simulink model "PCC_Calibration_Simu"  (R2015b)
settings: Solver=ode3  StartTime=0.0  StopTime=1373  FixedStep=0.01  RelTol=1e-3
model workspace: external: MAT-File params.mat (data not in the file)
undefined symbols (not defined in the file): aeroDragCoeff, airDensity, discIntervalf, discIntervals, DiscIntNeverNeededParam, FD, frontArea, G1, G2, G3, G4, G5, G6, gravity, inertialMassVeh, iterNum, lambdaRange, magnitude, massVeh, MDL, powerWeif, powerWeis, predPeriodf, predPeriods, rollingResistCoeff, terminThreshold, terminTimedis, terminVeloweif, terminVeloweis, wheelRadius, z_ACCe
libraries: simulink x16
(part 1 of 5)
settings Model: Creator=yanyongjun  LastModifiedBy=Administrator
settings DataIOCC: SaveFormat=Array
settings DebuggingCC: UnderspecifiedInitializationDetection=Classic  MergeDetectMultiDrivingBlocksExec=none  SolverPrmCheckMsg=warning  MultiTaskCondExecSysMsg=warning  MultiTaskRateTransMsg=warning
settings HardwareCC: ProdBitPerPointer=32  ProdLargestAtomicFloat=None  ProdIntDivRoundTo=Undefined  ProdEndianess=Unspecified  ProdWordSize=32  ProdHWDeviceType=32-bit Generic
settings GRTTargetCC: GeneratePreprocessorConditionals=Disable all
settings ConfigComp: CovModelRefEnable=Off

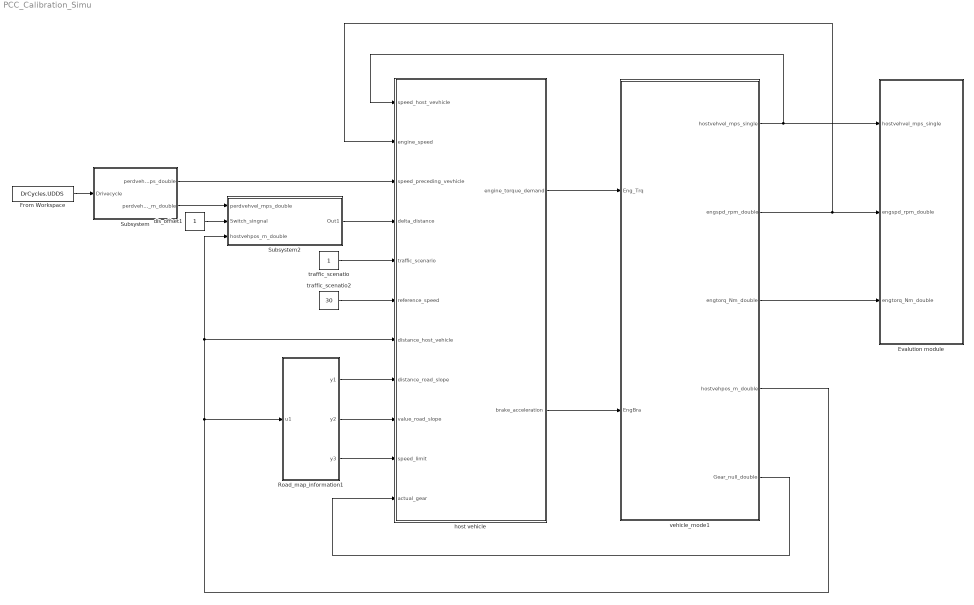
== system PCC_Calibration_Simu ==
  Evalution module : Subsystem
  From Workspace : FromWorkspace  VariableName=DrCycles.UDDS  SampleTime=0.01
  Road_map_information1 : MATLAB Function  TreatAsAtomicUnit=on
  Subsystem : Subsystem
  Subsystem2 : Subsystem
  dis_offset1 : Constant  OutDataTypeStr=double
  host vehicle : Subsystem
  traffic_scenatio : Constant  OutDataTypeStr=double
  traffic_scenatio2 : Constant  Value=30  OutDataTypeStr=double
  vehicle_mode1 : Subsystem
  wires:
  traffic_scenatio/1 -> host vehicle/5(traffic_scenario)
  Subsystem2/1(Out1) -> host vehicle/4(delta_distance)
  Subsystem/1(perdvehvel_mps_double) -> host vehicle/3(speed_preceding_vevhicle)
  traffic_scenatio2/1 -> host vehicle/6(reference_speed)
  vehicle_mode1/4(hostvehpos_m_double) -> Subsystem2/3(hostvehpos_m_double), host vehicle/7(distance_host_vehicle), Road_map_information1/1(u1)
  Road_map_information1/3(y3) -> host vehicle/10(speed_limit)
  Road_map_information1/2(y2) -> host vehicle/9(value_road_slope)
  host vehicle/1(engine_torque_demand) -> vehicle_mode1/1(Eng_Trq)
  Road_map_information1/1(y1) -> host vehicle/8(distance_road_slope)
  host vehicle/2(brake_acceleration) -> vehicle_mode1/2(EngBra)
  vehicle_mode1/5(Gear_null_double) -> host vehicle/11(actual_gear)
  vehicle_mode1/1(hostvehvel_mps_single) -> host vehicle/1(speed_host_vevhicle), Evalution module/1(hostvehvel_mps_single)
  From Workspace/1 -> Subsystem/1(Drivecycle)
  vehicle_mode1/3(engtorq_Nm_double) -> Evalution module/3(engtorq_Nm_double)
  Subsystem/2(perdvehpos_m_double) -> Subsystem2/1(perdvehvel_mps_double)
  dis_offset1/1 -> Subsystem2/2(Switch_singnal)
  vehicle_mode1/2(engspd_rpm_double) -> host vehicle/2(engine_speed), Evalution module/2(engspd_rpm_double)

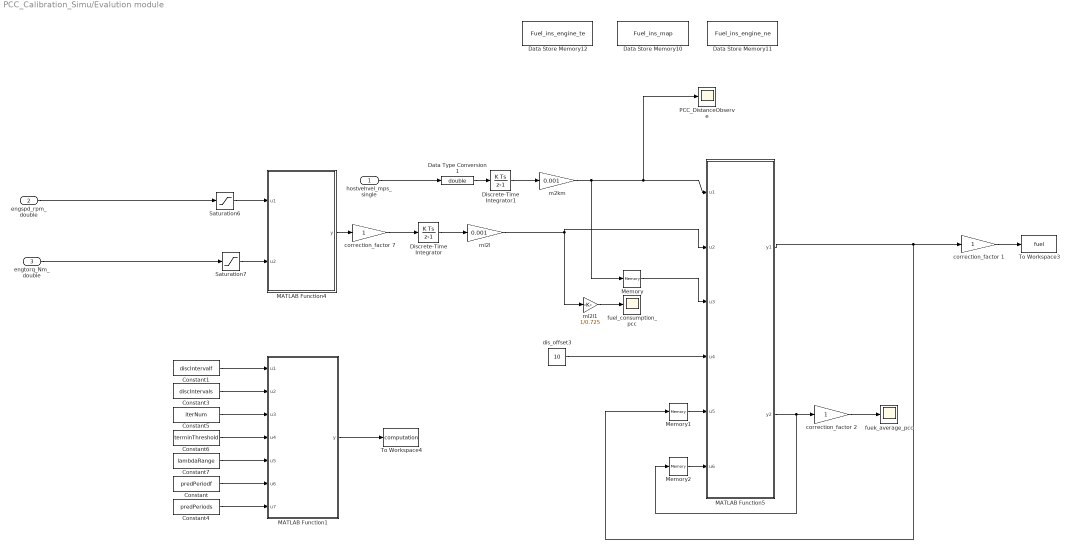
== system PCC_Calibration_Simu/Evalution module ==
  hostvehvel_mps_single : Inport
  engspd_rpm_double : Inport  Port=2
  engtorq_Nm_double : Inport  Port=3
  " ml2l" : Gain  Gain=0.001  SampleTime=0.01
  " ml2l1" : Gain  Gain=1/0.725  SampleTime=0.01
  Constant : Constant  Value=predPeriodf  OutDataTypeStr=double  SampleTime=0.01
  Constant1 : Constant  Value=discIntervalf  OutDataTypeStr=double  SampleTime=0.01
  Constant3 : Constant  Value=discIntervals  OutDataTypeStr=double  SampleTime=0.01
  Constant4 : Constant  Value=predPeriods  OutDataTypeStr=double  SampleTime=0.01
  Constant5 : Constant  Value=iterNum  OutDataTypeStr=double  SampleTime=0.01
  Constant6 : Constant  Value=terminThreshold  OutDataTypeStr=double  SampleTime=0.01
  Constant7 : Constant  Value=lambdaRange  OutDataTypeStr=double  SampleTime=0.01
  Data Store Memory10 : DataStoreMemory  DataStoreName=Fuel_ins_map  InitialValue=ones(21,111)  OutDataTypeStr=double
  Data Store Memory11 : DataStoreMemory  DataStoreName=Fuel_ins_engine_ne  InitialValue=ones(21,111)  OutDataTypeStr=double
  Data Store Memory12 : DataStoreMemory  DataStoreName=Fuel_ins_engine_te  InitialValue=ones(21,111)  OutDataTypeStr=double
  Data Type Conversion1 : DataTypeConversion  OutDataTypeStr=double
  Discrete-Time Integrator : DiscreteIntegrator  SampleTime=0.01  ICPrevOutput=DiscIntNeverNeededParam  ICPrevScaledInput=DiscIntNeverNeededParam
  Discrete-Time Integrator1 : DiscreteIntegrator  SampleTime=0.01  ICPrevOutput=DiscIntNeverNeededParam  ICPrevScaledInput=DiscIntNeverNeededParam
  MATLAB Function1 : MATLAB Function  TreatAsAtomicUnit=on
  MATLAB Function4 : MATLAB Function  TreatAsAtomicUnit=on
  MATLAB Function5 : MATLAB Function  TreatAsAtomicUnit=on
  Memory : Memory
  Memory1 : Memory
  Memory2 : Memory
  PCC_DistanceObserve : Scope
  Saturation6 : Saturate  UpperLimit=6500  LowerLimit=700
  Saturation7 : Saturate  UpperLimit=200  LowerLimit=-40
  To Workspace3 : ToWorkspace  VariableName=fuel  SampleTime=-1
  To Workspace4 : ToWorkspace  VariableName=computation  SampleTime=-1
  correction_factor 1 : Gain  SampleTime=0.01
  correction_factor 2 : Gain  SampleTime=0.01
  correction_factor 7 : Gain  SampleTime=0.01
  dis_offset3 : Constant  Value=10  OutDataTypeStr=double
  fuek_average_pcc : Scope
  fuel_consumption_pcc : Scope
  m2km : Gain  Gain=0.001  SampleTime=0.01
  wires:
  MATLAB Function5/1(y1) -> Memory1/1, correction_factor 1/1
  Memory/1 -> MATLAB Function5/3(u3)
  " ml2l"/1 -> MATLAB Function5/2(u2), " ml2l1"/1
  dis_offset3/1 -> MATLAB Function5/4(u4)
  Memory1/1 -> MATLAB Function5/5(u5)
  Memory2/1 -> MATLAB Function5/6(u6)
  m2km/1 -> Memory/1, PCC_DistanceObserve/1, MATLAB Function5/1(u1)
  engtorq_Nm_double/1 -> Saturation7/1
  correction_factor 1/1 -> To Workspace3/1
  Data Type Conversion1/1 -> Discrete-Time Integrator1/1
  MATLAB Function5/2(y2) -> Memory2/1, correction_factor 2/1
  hostvehvel_mps_single/1 -> Data Type Conversion1/1
  MATLAB Function4/1(y) -> correction_factor 7/1
  Discrete-Time Integrator/1 -> " ml2l"/1
  correction_factor 2/1 -> fuek_average_pcc/1
  Saturation6/1 -> MATLAB Function4/1(u1)
  correction_factor 7/1 -> Discrete-Time Integrator/1
  Discrete-Time Integrator1/1 -> m2km/1
  " ml2l1"/1 -> fuel_consumption_pcc/1
  Saturation7/1 -> MATLAB Function4/2(u2)
  engspd_rpm_double/1 -> Saturation6/1
  Constant1/1 -> MATLAB Function1/1(u1)
  MATLAB Function1/1(y) -> To Workspace4/1
  Constant5/1 -> MATLAB Function1/3(u3)
  Constant6/1 -> MATLAB Function1/4(u4)
  Constant7/1 -> MATLAB Function1/5(u5)
  Constant3/1 -> MATLAB Function1/2(u2)
  Constant/1 -> MATLAB Function1/6(u6)
  Constant4/1 -> MATLAB Function1/7(u7)

== system PCC_Calibration_Simu/Subsystem ==
  Drivecycle : Inport
  Add : Sum  Inputs=+-
  PID Controller : simulink/Continuous/PID Controller  Controller=PID  TimeDomain=Discrete-time  SampleTime=-1  IntegratorMethod=Forward Euler  FilterMethod=Forward Euler  Form=Parallel  UseFilter=on  ControllerParametersSource=internal  P=6  I=1  D=0  N=100  InitialConditionSource=internal  InitialConditionForIntegrator=0  InitialConditionForFilter=0  ExternalReset=none  LimitOutput=off  UpperSaturationLimit=inf  LowerSaturationLimit=-inf  LinearizeAsGain=on  AntiWindupMode=none  Kb=1  TrackingMode=off  Kt=1  PParamMin=[]  PParamMax=[]  IParamMin=[]  IParamMax=[]  DParamMin=[]  DParamMax=[]  NParamMin=[]  NParamMax=[]  KbParamMin=[]  KbParamMax=[]  KtParamMin=[]  KtParamMax=[]  POutMin=[]  POutMax=[]  IOutMin=[]  IOutMax=[]  DOutMin=[]  DOutMax=[]  NOutMin=[]  NOutMax=[]  KbOutMin=[]  KbOutMax=[]  KtOutMin=[]  KtOutMax=[]  IntegratorOutMin=[]  IntegratorOutMax=[]  FilterOutMin=[]  FilterOutMax=[]  SumOutMin=[]  SumOutMax=[]  SumI1OutMin=[]  SumI1OutMax=[]  SumI2OutMin=[]  SumI2OutMax=[]  SumI3OutMin=[]  SumI3OutMax=[]  SumDOutMin=[]  SumDOutMax=[]  SaturationOutMin=[]  SaturationOutMax=[]  IntegratorContinuousStateAttributes=''  IntegratorStateMustResolveToSignalObject=off  IntegratorRTWStateStorageClass=Auto  FilterContinuousStateAttributes=''  FilterStateMustResolveToSignalObject=off  FilterRTWStateStorageClass=Auto  DifferentiatorICPrevScaledInput=0  DifferentiatorOutMin=[]  DifferentiatorOutMax=[]
  Saturation2 : Saturate  UpperLimit=100  LowerLimit=0
  Saturation3 : Saturate  UpperLimit=0  LowerLimit=-100
  kmph2mps : Gain  Gain=1/3.6
  mph2kmph : Gain  Gain=1.6
  vehicle_mode : Subsystem
  perdvehvel_mps_double : Outport
  perdvehpos_m_double : Outport  Port=2
  wires:
  Drivecycle/1 -> Add/1
  kmph2mps/1 -> perdvehvel_mps_double/1
  Saturation2/1 -> vehicle_mode/1(Eng_Trq)
  Saturation3/1 -> vehicle_mode/2(EngBra)
  vehicle_mode/1(Position[m]) -> perdvehpos_m_double/1
  PID Controller/1 -> Saturation3/1, Saturation2/1
  vehicle_mode/2(Velocity[mph]) -> Add/2, mph2kmph/1
  mph2kmph/1 -> kmph2mps/1
  Add/1 -> PID Controller/1

== system PCC_Calibration_Simu/Subsystem2 ==
  perdvehvel_mps_double : Inport
  Switch_singnal : Inport  Port=2
  hostvehpos_m_double : Inport  Port=3
  Constant2 : Constant  Value=1000  OutDataTypeStr=double
  Subtract1 : Sum  Inputs=+-
  Sum : Sum  Inputs=|++
  Switch1 : Switch  Criteria=u2 > Threshold  Threshold=0.1
  To Workspace1 : ToWorkspace  VariableName=delta_dis  SampleTime=-1
  dis_offset2 : Constant  Value=3  OutDataTypeStr=double
  Out1 : Outport
  wires:
  Switch_singnal/1 -> Switch1/2
  dis_offset2/1 -> Sum/2
  Switch1/1 -> Out1/1
  Subtract1/1 -> Sum/1
  Constant2/1 -> Switch1/3
  Sum/1 -> To Workspace1/1, Switch1/1
  perdvehvel_mps_double/1 -> Subtract1/1
  hostvehpos_m_double/1 -> Subtract1/2

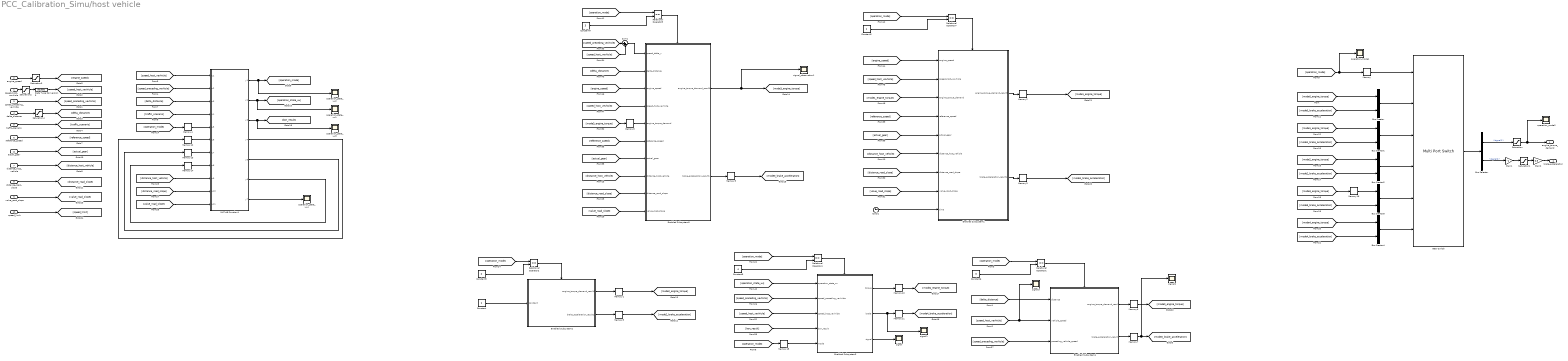
== system PCC_Calibration_Simu/host vehicle ==
  speed_host_vevhicle : Inport
  engine_speed : Inport  Port=2
  speed_preceding_vevhicle : Inport  Port=3
  delta_distance : Inport  Port=4
  traffic_scenario : Inport  Port=5
  reference_speed : Inport  Port=6
  distance_host_vehicle : Inport  Port=7
  distance_road_slope : Inport  Port=8
  value_road_slope : Inport  Port=9
  speed_limit : Inport  Port=10
  actual_gear : Inport  Port=11
  Bus Creator{,1..4} (5 alike) : BusCreator  Inputs=2
  Bus Selector : BusSelector  OutputSignals=signal1,signal2
  Clock1 : Clock
  Constant : Constant
  Constant2 : Constant
  Constant3 : Constant  Value=2
  Constant4 : Constant  Value=3
  Constant5 : Constant  Value=4
  Constant6 : Constant  Value=0
  Data Type Conversion3 : DataTypeConversion  OutDataTypeStr=double
  Enabled Subsystem1 : Subsystem  TreatAsAtomicUnit=on
  Enabled Subsystem2 : Subsystem  TreatAsAtomicUnit=on
  Enabled Subsystem3 : Subsystem  TreatAsAtomicUnit=on
  Enabled Subsystem4 : Subsystem  TreatAsAtomicUnit=on
  Enabled Subsystem5 : Subsystem  TreatAsAtomicUnit=on
  Gain1 : Gain  Gain=-1
  Gain2 : Gain  Gain=0.5
  Gear Switch : MultiPortSwitch  DataPortOrder=Zero-based contiguous  Inputs=5  zeroidx=on
  MATLAB Function1 : MATLAB Function  TreatAsAtomicUnit=on
  Memory{,1,3,5..7,9..11} (9 alike) : Memory
  Memory12 : Memory  X0=3
  Memory13 : Memory  X0=0.6
  Memory14 : Memory  X0=5
  Memory15 : Memory  X0=4
  Memory16 : Memory  X0=60
  Memory2 : Memory  X0=70
  Memory4 : Memory  X0=1
  Memory8 : Memory  X0=60
  Relational Operator{1..4,7} (5 alike) : RelationalOperator  Operator===  OutDataTypeStr=boolean
  Saturation : Saturate  UpperLimit=250  LowerLimit=-50
  Saturation1 : Saturate  UpperLimit=0  LowerLimit=-8
  Saturation2 : Saturate  UpperLimit=40  LowerLimit=0
  Saturation3 : Saturate  UpperLimit=7000  LowerLimit=500
  Saturation4 : Saturate  UpperLimit=1000  LowerLimit=0
  Sum1 : Sum  Inputs=|+-
  operation_mode1 : Scope
  operation_mode2 : Scope
  operation_state_uu{1..4} (4 alike) : Scope
  signal{,1..3} (4 alike) : Scope
  signal_observation1 : Scope
  engine_torque_demand : Outport
  brake_acceleration : Outport  Port=2
  wires:
  speed_host_vevhicle/1 -> Saturation2/1
  speed_preceding_vevhicle/1 -> [speed_preceding_vevhicle]
  delta_distance/1 -> Saturation4/1
  traffic_scenario/1 -> [traffic_scenario]
  engine_speed/1 -> Saturation3/1
  reference_speed/1 -> [reference_speed]
  Gain1/1 -> Saturation1/1
  Saturation/1 -> engine_torque_demand/1, operation_mode2/1
  Saturation1/1 -> Gain2/1
  Bus Creator/1 -> Gear Switch/2
  Gear Switch/1 -> Bus Selector/1
  Bus Selector/1 -> Saturation/1  "<signal1>"
  Bus Selector/2 -> Gain1/1  "<signal2>"
  Bus Creator1/1 -> Gear Switch/3
  Bus Creator2/1 -> Gear Switch/4
  Bus Creator3/1 -> Gear Switch/5
  Bus Creator4/1 -> Gear Switch/6
  Memory1/1 -> [mode2_engine_torque]
  Memory5/1 -> [mode2_brake_acceleration]
  Enabled Subsystem2/1(engine_torque_demand_result1) -> Memory1/1
  Enabled Subsystem2/2(brake_acceleration_result1) -> Memory5/1
  Constant/1 -> Enabled Subsystem2/1(constant)
  [operation_mode] -> Relational Operator2/1
  Relational Operator2/1 -> Enabled Subsystem2/Enable
  Constant3/1 -> Relational Operator2/2
  actual_gear/1 -> [actual_gear]
  [operation_mode] -> operation_mode1/1, Memory/1
  Memory/1 -> Gear Switch/1
  [engine_speed] -> Enabled Subsystem1/1(engine_speed)
  [reference_speed] -> Enabled Subsystem1/4(reference_speed)
  [operation_mode] -> Relational Operator7/1
  Relational Operator7/1 -> Enabled Subsystem1/Enable
  Constant2/1 -> Relational Operator7/2
  [actual_gear] -> Enabled Subsystem1/5(actual_gear)
  [speed_host_vevhicle] -> Enabled Subsystem1/2(speed_host_vevhicle)
  Enabled Subsystem3/1(torque) -> Memory10/1
  Enabled Subsystem3/2(brake) -> Memory11/1, signal1/1
  [operation_mode] -> Relational Operator4/1
  Relational Operator4/1 -> Enabled Subsystem3/Enable
  Constant5/1 -> Relational Operator4/2
  [operation_state_uu] -> Enabled Subsystem3/1(operation_state_uu)
  [speed_preceding_vevhicle] -> Enabled Subsystem3/2(speed_preceding_vevhicle)
  [speed_host_vevhicle] -> Enabled Subsystem3/3(speed_host_vevhicle)
  [bon_result] -> Enabled Subsystem3/4(bon_result)
  Memory10/1 -> [mode4_engine_torque]
  Memory11/1 -> [mode4_brake_acceleration]
  [speed_host_vevhicle] -> Sum1/2
  Sum1/1 -> Enabled Subsystem5/1(speed_delta_v)
  [delta_distance] -> Enabled Subsystem5/2(delta_distance)
  [engine_speed] -> Enabled Subsystem5/3(engine_speed)
  [speed_host_vevhicle] -> Enabled Subsystem5/4(speed_host_vevhicle)
  [mode3_engine_torque] -> Memory8/1
  [reference_speed] -> Enabled Subsystem5/6(reference_speed)
  [speed_preceding_vevhicle] -> Sum1/1
  Memory9/1 -> [mode3_brake_acceleration]
  Enabled Subsystem5/2(brake_acceleration_result1) -> Memory9/1
  [operation_mode] -> Relational Operator3/1
  Relational Operator3/1 -> Enabled Subsystem5/Enable
  Constant4/1 -> Relational Operator3/2
  [actual_gear] -> Enabled Subsystem5/7(actual_gear)
  Enabled Subsystem3/3(signal) -> signal/1
  Memory6/1 -> [mode0_engine_torque]
  Memory7/1 -> [mode0_brake_acceleration], signal2/1
  [operation_mode] -> Relational Operator1/1
  Relational Operator1/1 -> Enabled Subsystem4/Enable
  Constant6/1 -> Relational Operator1/2
  [operation_mode] -> Memory4/1
  MATLAB Function1/1(y1) -> operation_state_uu2/1, [operation_mode]
  MATLAB Function1/2(y2) -> operation_state_uu1/1, [operation_state_uu]
  [speed_host_vevhicle] -> MATLAB Function1/1(u1)
  [speed_preceding_vevhicle] -> MATLAB Function1/2(u2)
  [delta_distance] -> MATLAB Function1/3(u3)
  [traffic_scenario] -> MATLAB Function1/4(u4)
  MATLAB Function1/3(y3) -> operation_state_uu3/1, [bon_result]
  Memory4/1 -> MATLAB Function1/5(u5)
  MATLAB Function1/4(y4) -> Memory12/1
  MATLAB Function1/5(y5) -> Memory13/1
  Memory12/1 -> MATLAB Function1/6(u6)
  Memory13/1 -> MATLAB Function1/7(u7)
  Memory14/1 -> MATLAB Function1/8(u8)
  MATLAB Function1/6(y6) -> Memory14/1
  Enabled Subsystem1/1(engine_torque_demand_result1) -> Memory2/1
  Enabled Subsystem1/2(brake_acceleration_result1) -> Memory3/1
  [mode0_engine_torque] -> Bus Creator/1
  [mode1_engine_torque] -> Bus Creator1/1
  [mode0_brake_acceleration] -> Bus Creator/2
  [mode1_brake_acceleration] -> Bus Creator1/2
  [mode2_engine_torque] -> Bus Creator2/1
  [mode2_brake_acceleration] -> Bus Creator2/2
  [mode3_engine_torque] -> Memory16/1
  [mode3_brake_acceleration] -> Bus Creator3/2
  [mode4_engine_torque] -> Bus Creator4/1
  [mode4_brake_acceleration] -> Bus Creator4/2
  Memory2/1 -> [mode1_engine_torque]
  [mode1_engine_torque] -> Enabled Subsystem1/3(engine_torque_demand)
  Memory3/1 -> [mode1_brake_acceleration]
  [operation_mode] -> Memory15/1
  Memory15/1 -> Enabled Subsystem3/5(mode)
  Enabled Subsystem4/1(engine_torque_demand_result) -> Memory6/1
  Enabled Subsystem4/2(brake_acceleration_result) -> Memory7/1
  [delta_distance] -> Enabled Subsystem4/1(distance)
  [speed_preceding_vevhicle] -> Enabled Subsystem4/3(preceding_vehicle_speed)
  [speed_host_vevhicle] -> Enabled Subsystem4/2(vehicle_speed), signal3/1
  Memory8/1 -> Enabled Subsystem5/5(engine_torque_demand)
  Memory16/1 -> Bus Creator3/1
  Enabled Subsystem5/1(engine_torque_demand_result1) -> signal_observation1/1, [mode3_engine_torque]
  distance_host_vehicle/1 -> [distance_host_vehicle]
  [distance_host_vehicle] -> MATLAB Function1/9(u9)
  distance_road_slope/1 -> [distance_road_slope]
  [distance_road_slope] -> MATLAB Function1/10(u10)
  value_road_slope/1 -> [value_road_slope]
  [value_road_slope] -> MATLAB Function1/11(u11)
  speed_limit/1 -> [speed_limit]
  MATLAB Function1/7(y7) -> operation_state_uu4/1
  [distance_road_slope] -> Enabled Subsystem5/9(distance_road_slope)
  [value_road_slope] -> Enabled Subsystem5/10(value_road_slope)
  [distance_host_vehicle] -> Enabled Subsystem5/8(distance_host_vehicle)
  [distance_road_slope] -> Enabled Subsystem1/7(distance_road_slope)
  [value_road_slope] -> Enabled Subsystem1/8(value_road_slope)
  [distance_host_vehicle] -> Enabled Subsystem1/6(distance_host_vehicle)
  Clock1/1 -> Enabled Subsystem1/9(time)
  Saturation2/1 -> Data Type Conversion3/1
  Data Type Conversion3/1 -> [speed_host_vevhicle]
  Saturation3/1 -> [engine_speed]
  Saturation4/1 -> [delta_distance]
  Gain2/1 -> brake_acceleration/1

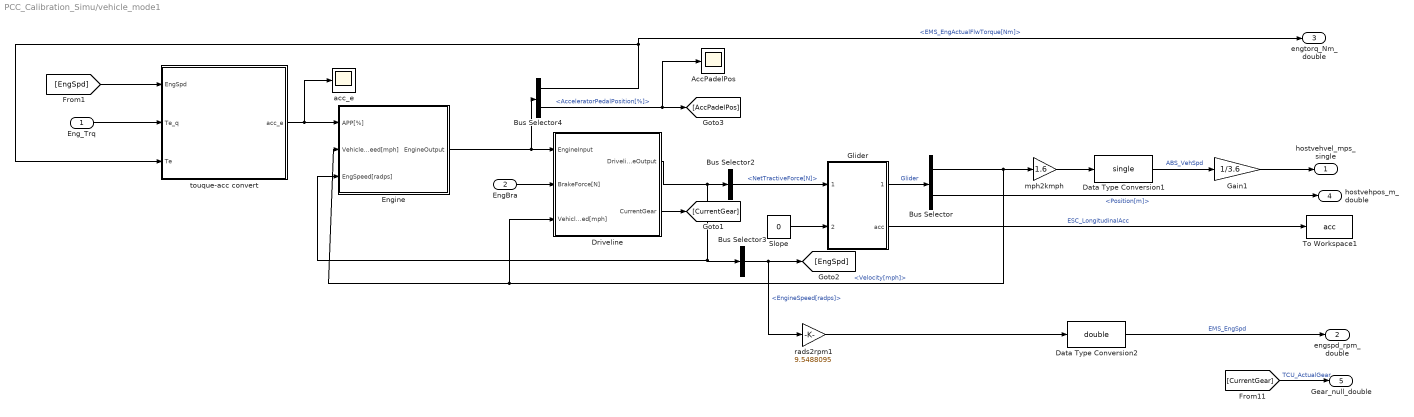
== system PCC_Calibration_Simu/vehicle_mode1 ==
  Eng_Trq : Inport
  EngBra : Inport  Port=2
  AccPadelPos : Scope
  Bus Selector : BusSelector  OutputSignals=Velocity[mph],Position[m]
  Bus Selector2 : BusSelector  OutputSignals=NetTractiveForce[N]
  Bus Selector3 : BusSelector  OutputSignals=EngineSpeed[radps]
  Bus Selector4 : BusSelector  OutputSignals=EMS_EngActualFlwTorque[Nm],AcceleratorPedalPosition[%]
  Data Type Conversion1 : DataTypeConversion  OutDataTypeStr=single
  Data Type Conversion2 : DataTypeConversion  OutDataTypeStr=double
  Driveline : Subsystem
      settings: MinAlgLoopOccurrences=on
      mask Display: image(imread('driveline.jpg'));
  Engine : Subsystem
      mask Display: image('engine.jpg');
  Gain1 : Gain  Gain=1/3.6
  Glider : Subsystem  AncestorBlock=Driver_Glider_Library/Glider
      mask Display: image(imread('DriverPic.jpg'))
  Slope : Constant  Value=0
  To Workspace1 : ToWorkspace  VariableName=acc  SampleTime=-1
  acc_e : Scope
  mph2kmph : Gain  Gain=1.6
  rads2rpm1 : Gain  Gain=9.5488095
  touque-acc convert : Subsystem
      settings: MinAlgLoopOccurrences=on
  hostvehvel_mps_single : Outport
  engspd_rpm_double : Outport  Port=2
  engtorq_Nm_double : Outport  Port=3
  hostvehpos_m_double : Outport  Port=4
  Gear_null_double : Outport  Port=5
  wires:
  Driveline/2(CurrentGear) -> [CurrentGear]
  Bus Selector4/2 -> [AccPadelPos], AccPadelPos/1  "<AcceleratorPedalPosition[%]>"
  rads2rpm1/1 -> Data Type Conversion2/1
  mph2kmph/1 -> Data Type Conversion1/1
  Slope/1 -> Glider/2(slope_angle[°])
  Bus Selector4/1 -> engtorq_Nm_double/1, touque-acc convert/3(Te)  "<EMS_EngActualFlwTorque[Nm]>"
  Bus Selector3/1 -> [EngSpd], rads2rpm1/1  "<EngineSpeed[radps]>"
  Bus Selector2/1 -> Glider/1(tractiveForce[N])  "<NetTractiveForce[N]>"
  Bus Selector/1 -> Driveline/3(VehicleSpeed[mph]), Engine/2(VehicleSpeed[mph]), mph2kmph/1  "<Velocity[mph]>"
  EngBra/1 -> Driveline/2(BrakeForce[N])
  Driveline/1(DrivelineOutput) -> Bus Selector3/1, Engine/3(EngSpeed[radps]), Bus Selector2/1
  Engine/1(EngineOutput) -> Driveline/1(EngineInput), Bus Selector4/1
  touque-acc convert/1(acc_e) -> Engine/1(APP[%]), acc_e/1
  Glider/1(GliderOutput) -> Bus Selector/1  "Glider"
  Eng_Trq/1 -> touque-acc convert/2(Te_q)
  [EngSpd] -> touque-acc convert/1(EngSpd)
  Data Type Conversion2/1 -> engspd_rpm_double/1  "EMS_EngSpd"
  Data Type Conversion1/1 -> Gain1/1  "ABS_VehSpd"
  [CurrentGear] -> Gear_null_double/1  "TCU_ActualGear"
  Bus Selector/2 -> hostvehpos_m_double/1  "<Position[m]>"
  Glider/2(acc) -> To Workspace1/1  "ESC_LongitudinalAcc"
  Gain1/1 -> hostvehvel_mps_single/1

== system PCC_Calibration_Simu/Subsystem/vehicle_mode ==
  Eng_Trq : Inport
  EngBra : Inport  Port=2
  Bus Selector : BusSelector  OutputSignals=Velocity[mph],Position[m]
  Bus Selector2 : BusSelector  OutputSignals=NetTractiveForce[N]
  Bus Selector3 : BusSelector  OutputSignals=EngineSpeed[radps]
  Driveline : Subsystem
      settings: MinAlgLoopOccurrences=on
      mask Display: image(imread('driveline.jpg'));
  Engine : Subsystem
      mask Display: image('engine.jpg');
  Glider : Subsystem  AncestorBlock=Driver_Glider_Library/Glider
      mask Display: image(imread('DriverPic.jpg'))
  Scope2 : Scope
  Slope : Constant  Value=0
  mph2kmph1 : Gain  Gain=1.6
  Position[m] : Outport
  Velocity[mph] : Outport  Port=2
  wires:
  Glider/1(GliderOutput) -> Bus Selector/1  "Glider"
  Engine/1(EngineOutput) -> Driveline/1(EngineInput)
  Driveline/1(DrivelineOutput) -> Bus Selector2/1, Engine/3(EngSpeed[radps]), Bus Selector3/1
  EngBra/1 -> Driveline/2(BrakeForce[N])
  Bus Selector/1 -> Velocity[mph]/1, Engine/2(VehicleSpeed[mph]), Driveline/3(VehicleSpeed[mph]), mph2kmph1/1  "<Velocity[mph]>"
  Bus Selector2/1 -> Glider/1(tractiveForce[N])  "<NetTractiveForce[N]>"
  Bus Selector3/1 -> [EngSpd]  "<EngineSpeed[radps]>"
  Slope/1 -> Glider/2(slope_angle[°])
  mph2kmph1/1 -> Scope2/1  "Velocity[mps]"
  Driveline/2(CurrentGear) -> [CurrentGear]
  Eng_Trq/1 -> Engine/1(APP[%])
  Bus Selector/2 -> Position[m]/1  "<Position[m]>"

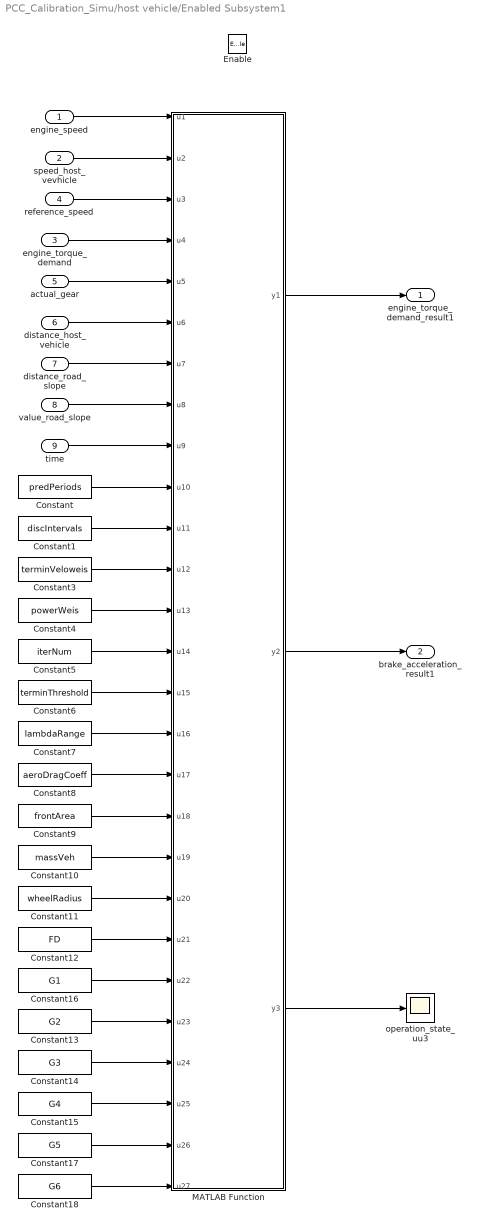
== system PCC_Calibration_Simu/host vehicle/Enabled Subsystem1 ==
  engine_speed : Inport
  speed_host_vevhicle : Inport  Port=2
  engine_torque_demand : Inport  Port=3
  reference_speed : Inport  Port=4
  actual_gear : Inport  Port=5
  distance_host_vehicle : Inport  Port=6
  distance_road_slope : Inport  Port=7
  value_road_slope : Inport  Port=8
  time : Inport  Port=9
  Enable : EnablePort
  Constant : Constant  Value=predPeriods  OutDataTypeStr=double  SampleTime=0.01
  Constant1 : Constant  Value=discIntervals  OutDataTypeStr=double  SampleTime=0.01
  Constant10 : Constant  Value=massVeh  OutDataTypeStr=double  SampleTime=0.01
  Constant11 : Constant  Value=wheelRadius  OutDataTypeStr=double  SampleTime=0.01
  Constant12 : Constant  Value=FD  OutDataTypeStr=double  SampleTime=0.01
  Constant13 : Constant  Value=G2  OutDataTypeStr=double  SampleTime=0.01
  Constant14 : Constant  Value=G3  OutDataTypeStr=double  SampleTime=0.01
  Constant15 : Constant  Value=G4  OutDataTypeStr=double  SampleTime=0.01
  Constant16 : Constant  Value=G1  OutDataTypeStr=double  SampleTime=0.01
  Constant17 : Constant  Value=G5  OutDataTypeStr=double  SampleTime=0.01
  Constant18 : Constant  Value=G6  OutDataTypeStr=double  SampleTime=0.01
  Constant3 : Constant  Value=terminVeloweis  OutDataTypeStr=double  SampleTime=0.01
  Constant4 : Constant  Value=powerWeis  OutDataTypeStr=double  SampleTime=0.01
  Constant5 : Constant  Value=iterNum  OutDataTypeStr=double  SampleTime=0.01
  Constant6 : Constant  Value=terminThreshold  OutDataTypeStr=double  SampleTime=0.01
  Constant7 : Constant  Value=lambdaRange  OutDataTypeStr=double  SampleTime=0.01
  Constant8 : Constant  Value=aeroDragCoeff  OutDataTypeStr=double  SampleTime=0.01
  Constant9 : Constant  Value=frontArea  OutDataTypeStr=double  SampleTime=0.01
  MATLAB Function : MATLAB Function  TreatAsAtomicUnit=on
  operation_state_uu3 : Scope
  engine_torque_demand_result1 : Outport
  brake_acceleration_result1 : Outport  Port=2
  wires:
  MATLAB Function/1(y1) -> engine_torque_demand_result1/1
  MATLAB Function/2(y2) -> brake_acceleration_result1/1
  engine_speed/1 -> MATLAB Function/1(u1)
  speed_host_vevhicle/1 -> MATLAB Function/2(u2)
  reference_speed/1 -> MATLAB Function/3(u3)
  engine_torque_demand/1 -> MATLAB Function/4(u4)
  actual_gear/1 -> MATLAB Function/5(u5)
  distance_host_vehicle/1 -> MATLAB Function/6(u6)
  distance_road_slope/1 -> MATLAB Function/7(u7)
  value_road_slope/1 -> MATLAB Function/8(u8)
  time/1 -> MATLAB Function/9(u9)
  MATLAB Function/3(y3) -> operation_state_uu3/1
  Constant/1 -> MATLAB Function/10(u10)
  Constant1/1 -> MATLAB Function/11(u11)
  Constant3/1 -> MATLAB Function/12(u12)
  Constant4/1 -> MATLAB Function/13(u13)
  Constant5/1 -> MATLAB Function/14(u14)
  Constant6/1 -> MATLAB Function/15(u15)
  Constant7/1 -> MATLAB Function/16(u16)
  Constant8/1 -> MATLAB Function/17(u17)
  Constant9/1 -> MATLAB Function/18(u18)
  Constant10/1 -> MATLAB Function/19(u19)
  Constant11/1 -> MATLAB Function/20(u20)
  Constant12/1 -> MATLAB Function/21(u21)
  Constant16/1 -> MATLAB Function/22(u22)
  Constant13/1 -> MATLAB Function/23(u23)
  Constant14/1 -> MATLAB Function/24(u24)
  Constant15/1 -> MATLAB Function/25(u25)
  Constant17/1 -> MATLAB Function/26(u26)
  Constant18/1 -> MATLAB Function/27(u27)

== system PCC_Calibration_Simu/host vehicle/Enabled Subsystem2 ==
  constant : Inport
  Enable : EnablePort
  Constant : Constant  Value=0
  Constant1 : Constant  Value=0
  engine_torque_demand_result1 : Outport
  brake_acceleration_result1 : Outport  Port=2
  wires:
  Constant/1 -> engine_torque_demand_result1/1
  Constant1/1 -> brake_acceleration_result1/1

== system PCC_Calibration_Simu/host vehicle/Enabled Subsystem3 ==
  operation_state_uu : Inport
  speed_preceding_vevhicle : Inport  Port=2
  speed_host_vevhicle : Inport  Port=3
  bon_result : Inport  Port=4
  mode : Inport  Port=5
  Enable : EnablePort
  Constant2 : Constant  Value=0
  MATLAB Function : MATLAB Function  TreatAsAtomicUnit=on
  Memory1 : Memory  X0=10
  Memory10 : Memory  X0=0.5
  torque : Outport
  brake : Outport  Port=2
  signal : Outport  Port=3
  wires:
  Constant2/1 -> torque/1
  operation_state_uu/1 -> MATLAB Function/1(u1)
  MATLAB Function/1(y1) -> brake/1
  speed_preceding_vevhicle/1 -> MATLAB Function/2(u2)
  speed_host_vevhicle/1 -> MATLAB Function/3(u3)
  bon_result/1 -> MATLAB Function/4(u4)
  MATLAB Function/2(y2) -> signal/1, Memory10/1
  Memory10/1 -> MATLAB Function/6(u6)
  mode/1 -> MATLAB Function/5(u5)
  Memory1/1 -> MATLAB Function/7(u7)
  MATLAB Function/3(y3) -> Memory1/1

== system PCC_Calibration_Simu/host vehicle/Enabled Subsystem4 ==
  distance : Inport
  vehicle_speed : Inport  Port=2
  preceding_vehicle_speed : Inport  Port=3
  Enable : EnablePort
  MATLAB Function : MATLAB Function  TreatAsAtomicUnit=on
  Memory : Memory  X0=2
  Memory1 : Memory
  Memory2 : Memory
  signal{1..4,10} (5 alike) : Scope
  engine_torque_demand_result : Outport
  brake_acceleration_result : Outport  Port=2
  wires:
  vehicle_speed/1 -> MATLAB Function/2(u2)
  preceding_vehicle_speed/1 -> MATLAB Function/3(u3)
  MATLAB Function/1(y1) -> engine_torque_demand_result/1, signal10/1
  MATLAB Function/2(y2) -> Memory2/1, brake_acceleration_result/1, signal1/1
  MATLAB Function/3(y3) -> Memory/1
  Memory/1 -> MATLAB Function/4(u4), signal2/1
  MATLAB Function/4(y4) -> Memory1/1
  Memory2/1 -> MATLAB Function/5(u5)
  Memory1/1 -> MATLAB Function/6(u6), signal3/1
  distance/1 -> MATLAB Function/1(u1), signal4/1

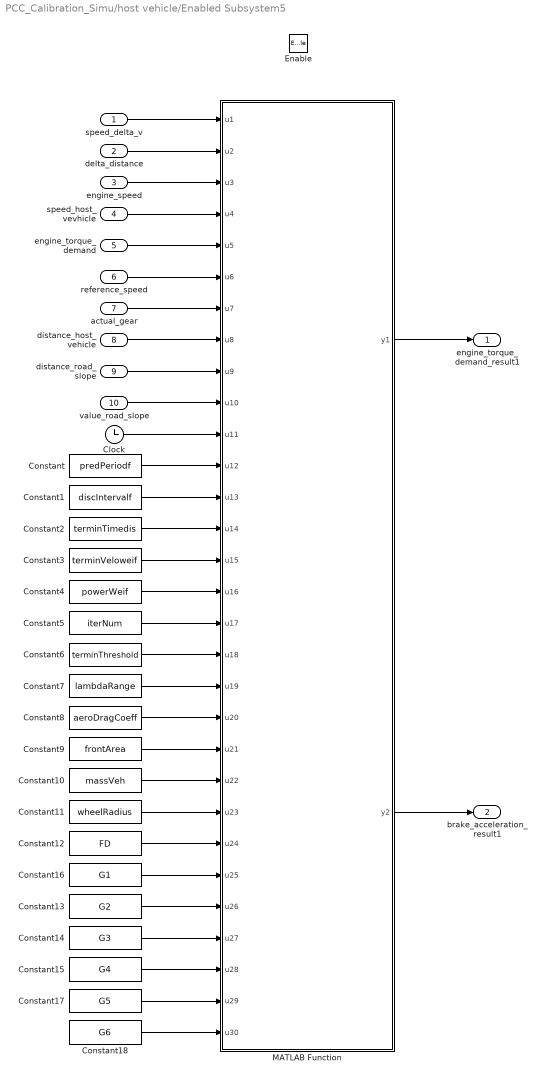
== system PCC_Calibration_Simu/host vehicle/Enabled Subsystem5 ==
  speed_delta_v : Inport
  delta_distance : Inport  Port=2
  engine_speed : Inport  Port=3
  speed_host_vevhicle : Inport  Port=4
  engine_torque_demand : Inport  Port=5
  reference_speed : Inport  Port=6
  actual_gear : Inport  Port=7
  distance_host_vehicle : Inport  Port=8
  distance_road_slope : Inport  Port=9
  value_road_slope : Inport  Port=10
  Enable : EnablePort
  Clock : Clock
  Constant : Constant  Value=predPeriodf  OutDataTypeStr=double  SampleTime=0.01
  Constant1 : Constant  Value=discIntervalf  OutDataTypeStr=double  SampleTime=0.01
  Constant10 : Constant  Value=massVeh  OutDataTypeStr=double  SampleTime=0.01
  Constant11 : Constant  Value=wheelRadius  OutDataTypeStr=double  SampleTime=0.01
  Constant12 : Constant  Value=FD  OutDataTypeStr=double  SampleTime=0.01
  Constant13 : Constant  Value=G2  OutDataTypeStr=double  SampleTime=0.01
  Constant14 : Constant  Value=G3  OutDataTypeStr=double  SampleTime=0.01
  Constant15 : Constant  Value=G4  OutDataTypeStr=double  SampleTime=0.01
  Constant16 : Constant  Value=G1  OutDataTypeStr=double  SampleTime=0.01
  Constant17 : Constant  Value=G5  OutDataTypeStr=double  SampleTime=0.01
  Constant18 : Constant  Value=G6  OutDataTypeStr=double  SampleTime=0.01
  Constant2 : Constant  Value=terminTimedis  OutDataTypeStr=double  SampleTime=0.01
  Constant3 : Constant  Value=terminVeloweif  OutDataTypeStr=double  SampleTime=0.01
  Constant4 : Constant  Value=powerWeif  OutDataTypeStr=double  SampleTime=0.01
  Constant5 : Constant  Value=iterNum  OutDataTypeStr=double  SampleTime=0.01
  Constant6 : Constant  Value=terminThreshold  OutDataTypeStr=double  SampleTime=0.01
  Constant7 : Constant  Value=lambdaRange  OutDataTypeStr=double  SampleTime=0.01
  Constant8 : Constant  Value=aeroDragCoeff  OutDataTypeStr=double  SampleTime=0.01
  Constant9 : Constant  Value=frontArea  OutDataTypeStr=double  SampleTime=0.01
  MATLAB Function : MATLAB Function  TreatAsAtomicUnit=on
  engine_torque_demand_result1 : Outport
  brake_acceleration_result1 : Outport  Port=2
  wires:
  speed_delta_v/1 -> MATLAB Function/1(u1)
  delta_distance/1 -> MATLAB Function/2(u2)
  engine_speed/1 -> MATLAB Function/3(u3)
  speed_host_vevhicle/1 -> MATLAB Function/4(u4)
  MATLAB Function/1(y1) -> engine_torque_demand_result1/1
  MATLAB Function/2(y2) -> brake_acceleration_result1/1
  engine_torque_demand/1 -> MATLAB Function/5(u5)
  reference_speed/1 -> MATLAB Function/6(u6)
  actual_gear/1 -> MATLAB Function/7(u7)
  distance_host_vehicle/1 -> MATLAB Function/8(u8)
  distance_road_slope/1 -> MATLAB Function/9(u9)
  value_road_slope/1 -> MATLAB Function/10(u10)
  Clock/1 -> MATLAB Function/11(u11)
  Constant/1 -> MATLAB Function/12(u12)
  Constant1/1 -> MATLAB Function/13(u13)
  Constant2/1 -> MATLAB Function/14(u14)
  Constant3/1 -> MATLAB Function/15(u15)
  Constant4/1 -> MATLAB Function/16(u16)
  Constant5/1 -> MATLAB Function/17(u17)
  Constant6/1 -> MATLAB Function/18(u18)
  Constant7/1 -> MATLAB Function/19(u19)
  Constant8/1 -> MATLAB Function/20(u20)
  Constant9/1 -> MATLAB Function/21(u21)
  Constant10/1 -> MATLAB Function/22(u22)
  Constant11/1 -> MATLAB Function/23(u23)
  Constant12/1 -> MATLAB Function/24(u24)
  Constant16/1 -> MATLAB Function/25(u25)
  Constant15/1 -> MATLAB Function/28(u28)
  Constant13/1 -> MATLAB Function/26(u26)
  Constant14/1 -> MATLAB Function/27(u27)
  Constant17/1 -> MATLAB Function/29(u29)
  Constant18/1 -> MATLAB Function/30(u30)

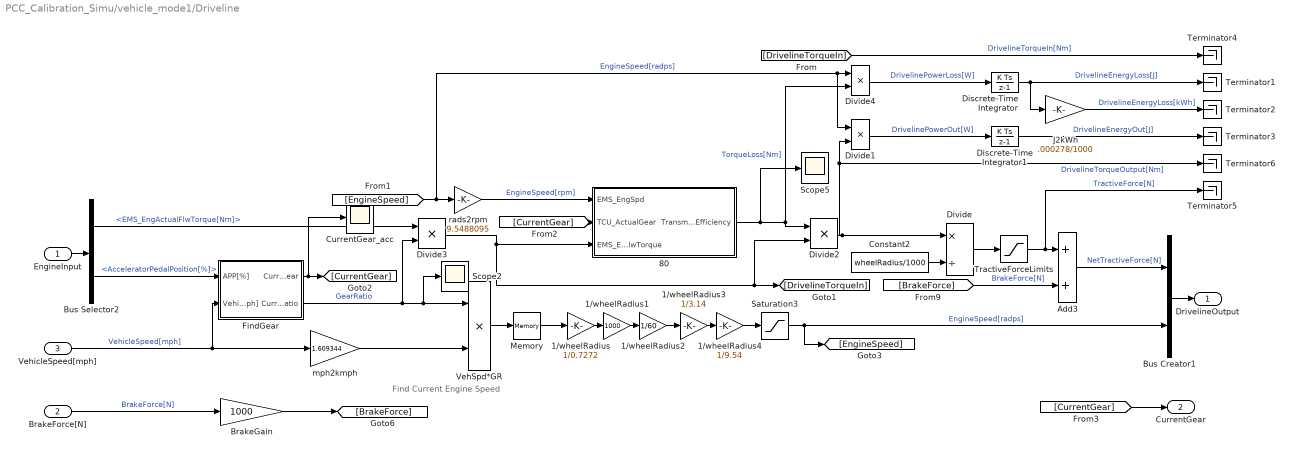
== system PCC_Calibration_Simu/vehicle_mode1/Driveline ==
  note: Find Current Engine Speed
  EngineInput : Inport
  BrakeForce[N] : Inport  Port=2
  VehicleSpeed[mph] : Inport  Port=3
  1/wheelRadius : Gain  Gain=1/0.7272
  1/wheelRadius1 : Gain  Gain=1000
  1/wheelRadius2 : Gain  Gain=1/60
  1/wheelRadius3 : Gain  Gain=1/3.14
  1/wheelRadius4 : Gain  Gain=1/9.54
  80 : Subsystem
  Add3 : Sum
  BrakeGain : Gain  Gain=1000
  Bus Creator1 : BusCreator  Inputs=2
  Bus Selector2 : BusSelector  OutputSignals=EMS_EngActualFlwTorque[Nm],AcceleratorPedalPosition[%]
  Constant2 : Constant  Value=wheelRadius/1000
  CurrentGear_acc : Scope
  Discrete-Time Integrator : DiscreteIntegrator  SampleTime=0.01  ICPrevOutput=DiscIntNeverNeededParam  ICPrevScaledInput=DiscIntNeverNeededParam
  Discrete-Time Integrator1 : DiscreteIntegrator  SampleTime=0.01  ICPrevOutput=DiscIntNeverNeededParam  ICPrevScaledInput=DiscIntNeverNeededParam
  Divide : Product  Inputs=*/
  Divide{1..4} (4 alike) : Product  Inputs=**
  FindGear : Subsystem
  J2kWh : Gain  Gain=.000278/1000
  Memory : Memory  InheritSampleTime=on
  Saturation3 : Saturate  UpperLimit=inf  LowerLimit=0.001  ZeroCross=off
  Scope2 : Scope
  Scope5 : Scope
  Terminator{1..6} (6 alike) : Terminator
  TractiveForceLimits : Saturate  UpperLimit=MDL.DrivelineModel.Ftr_max  LowerLimit=0  ZeroCross=off
  VehSpd*GR : Product  Inputs=**
  mph2kmph : Gain  Gain=1.609344
  rads2rpm : Gain  Gain=9.5488095
  DrivelineOutput : Outport
  CurrentGear : Outport  Port=2
  wires:
  Memory/1 -> 1/wheelRadius/1
  VehSpd*GR/1 -> Memory/1
  [CurrentGear] -> CurrentGear/1
  1/wheelRadius4/1 -> Saturation3/1
  1/wheelRadius3/1 -> 1/wheelRadius4/1
  1/wheelRadius2/1 -> 1/wheelRadius3/1
  1/wheelRadius1/1 -> 1/wheelRadius2/1
  mph2kmph/1 -> VehSpd*GR/2
  1/wheelRadius/1 -> 1/wheelRadius1/1
  [CurrentGear] -> 80/2(TCU_ActualGear)
  FindGear/1(CurrentGear) -> [CurrentGear], CurrentGear_acc/1
  BrakeGain/1 -> [BrakeForce]
  VehicleSpeed[mph]/1 -> FindGear/2(VehicleSpeed[mph]), mph2kmph/1  "VehicleSpeed[mph]"
  BrakeForce[N]/1 -> BrakeGain/1  "BrakeForce[N]"
  [DrivelineTorqueIn] -> Terminator4/1  "DrivelineTorqueIn[Nm]"
  Bus Creator1/1 -> DrivelineOutput/1
  rads2rpm/1 -> 80/1(EMS_EngSpd)  "EngineSpeed[rpm]"
  80/1(TransmissionEfficiency) -> Divide2/1, Divide4/2, Scope5/1  "TorqueLoss[Nm]"
  Bus Selector2/2 -> FindGear/1(APP[%])  "<AcceleratorPedalPosition[%]>"
  Discrete-Time Integrator/1 -> Terminator1/1, J2kWh/1  "DrivelineEnergyLoss[J]"
  J2kWh/1 -> Terminator2/1  "DrivelineEnergyLoss[kWh]"
  Discrete-Time Integrator1/1 -> Terminator3/1  "DrivelineEnergyOut[J]"
  Divide1/1 -> Discrete-Time Integrator1/1  "DrivelinePowerOut[W]"
  [EngineSpeed] -> Divide4/1, Divide1/1, rads2rpm/1  "EngineSpeed[radps]"
  Divide4/1 -> Discrete-Time Integrator/1  "DrivelinePowerLoss[W]"
  Divide3/1 -> [DrivelineTorqueIn], Divide2/2, 80/3(EMS_EngActualFlwTorque)
  Bus Selector2/1 -> Divide3/1  "<EMS_EngActualFlwTorque[Nm]>"
  Constant2/1 -> Divide/2
  FindGear/2(CurrentGearRatio) -> VehSpd*GR/1, Scope2/1, Divide3/2  "GearRatio"
  Saturation3/1 -> Bus Creator1/2, [EngineSpeed]  "EngineSpeed[radps]"
  Add3/1 -> Bus Creator1/1  "NetTractiveForce[N]"
  EngineInput/1 -> Bus Selector2/1
  TractiveForceLimits/1 -> Add3/1, Terminator5/1  "TractiveForce[N]"
  [BrakeForce] -> Add3/2  "BrakeForce[N]"
  Divide/1 -> TractiveForceLimits/1
  Divide2/1 -> Divide/1, Divide1/2, Terminator6/1  "DrivelineTorqueOutput[Nm]"

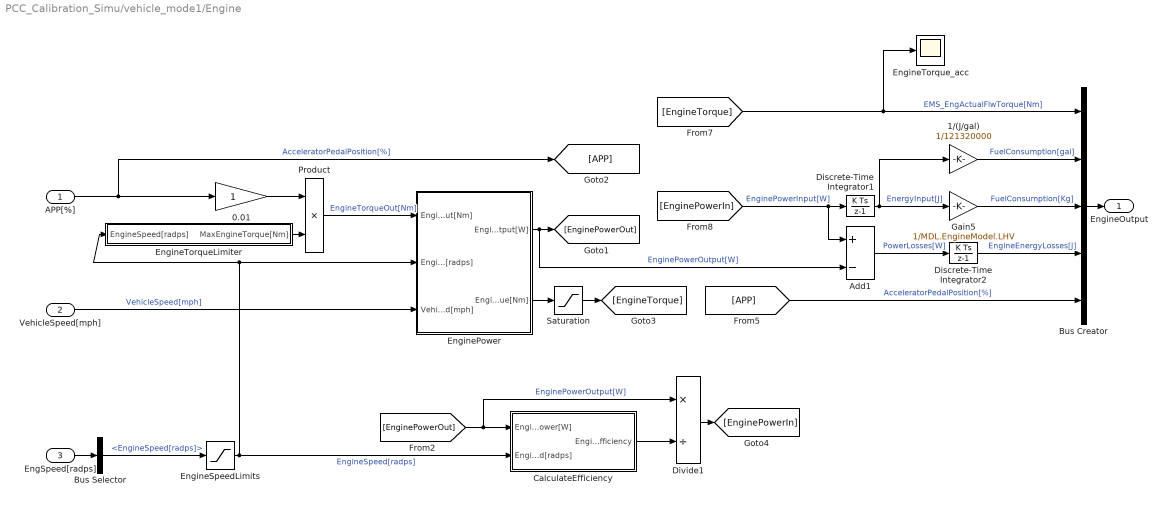
== system PCC_Calibration_Simu/vehicle_mode1/Engine ==
  APP[%] : Inport
  VehicleSpeed[mph] : Inport  Port=2
  EngSpeed[radps] : Inport  Port=3
  0.01 : Gain
  1/(J/gal) : Gain  Gain=1/121320000
  Add1 : Sum  Inputs=+-
  Bus Creator : BusCreator  Inputs=5
  Bus Selector : BusSelector  OutputSignals=EngineSpeed[radps]
  CalculateEfficiency : Subsystem
  Discrete-Time Integrator1 : DiscreteIntegrator  SampleTime=0.01  ICPrevOutput=DiscIntNeverNeededParam  ICPrevScaledInput=DiscIntNeverNeededParam
  Discrete-Time Integrator2 : DiscreteIntegrator  SampleTime=0.01  ICPrevOutput=DiscIntNeverNeededParam  ICPrevScaledInput=DiscIntNeverNeededParam
  Divide1 : Product  Inputs=*/
  EnginePower : Subsystem
  EngineSpeedLimits : Saturate  UpperLimit=940  LowerLimit=84
  EngineTorqueLimiter : Subsystem
  EngineTorque_acc : Scope
  Gain5 : Gain  Gain=1/MDL.EngineModel.LHV
      settings: AttributesFormatString=%<Gain>
  Product : Product  RndMeth=Zero
  Saturation : Saturate  UpperLimit=120  LowerLimit=0
  EngineOutput : Outport
  wires:
  Saturation/1 -> [EngineTorque]
  [EnginePowerIn] -> Add1/1, Discrete-Time Integrator1/1  "EnginePowerInput[W]"
  Divide1/1 -> [EnginePowerIn]
  [EngineTorque] -> Bus Creator/1, EngineTorque_acc/1  "EMS_EngActualFlwTorque[Nm]"
  EnginePower/2(EngineTorque[Nm]) -> Saturation/1
  EnginePower/1(EnginePowerOutput[W]) -> Add1/2, [EnginePowerOut]  "EnginePowerOutput[W]"
  [EnginePowerOut] -> CalculateEfficiency/1(EnginePower[W]), Divide1/1  "EnginePowerOutput[W]"
  Bus Selector/1 -> EngineSpeedLimits/1  "<EngineSpeed[radps]>"
  VehicleSpeed[mph]/1 -> EnginePower/3(VehicleSpeed[mph])  "VehicleSpeed[mph]"
  EngineSpeedLimits/1 -> CalculateEfficiency/2("EngineSpeed[radps] "), EngineTorqueLimiter/1(EngineSpeed[radps]), EnginePower/2(EngineSpeed[radps])  "EngineSpeed[radps]"
  Product/1 -> EnginePower/1(EngineTorqueOut[Nm])  "EngineTorqueOut[Nm]"
  EngineTorqueLimiter/1(MaxEngineTorque[Nm]) -> Product/2
  [APP] -> Bus Creator/5  "AcceleratorPedalPosition[%]"
  Add1/1 -> Discrete-Time Integrator2/1  "PowerLosses[W]"
  CalculateEfficiency/1(EngineEfficiency) -> Divide1/2
  EngSpeed[radps]/1 -> Bus Selector/1
  Gain5/1 -> Bus Creator/3  "FuelConsumption[Kg]"
  Discrete-Time Integrator2/1 -> Bus Creator/4  "EngineEnergyLosses[J]"
  1/(J/gal)/1 -> Bus Creator/2  "FuelConsumption[gal]"
  Bus Creator/1 -> EngineOutput/1
  Discrete-Time Integrator1/1 -> 1/(J/gal)/1, Gain5/1  "EnergyInput[J]"
  0.01/1 -> Product/1
  APP[%]/1 -> 0.01/1, [APP]  "AcceleratorPedalPosition[%]"

== system PCC_Calibration_Simu/vehicle_mode1/Glider ==
  note: F_g_r_a_d_e = m g sin(\theta)
  note: F_a_e_r_o = 1/2 \rho C_d A_f V ^2
  note: For Analysis & Results
  note: F_r_r = m g C_r_r
  note: a = (F_t_r - F_a_e_r_o - F_g_r_a_d_e - F_r_r) \div m_i
  note: F_t_r = F_a_e_r_o + F_i + F_g_r_a_d_e + F_r_r
  tractiveForce[N] : Inport
  slope_angle[°] : Inport  Port=2
  AerodynamicDrag[N] : Gain  Gain=0.5*airDensity*aeroDragCoeff*frontArea
      settings: AttributesFormatString=%<Gain>
  AerodynamicDrag[N]1 : Gain  Gain=1.6
      settings: AttributesFormatString=%<Gain>
  Bus Creator : BusCreator  Inputs=7
  Discrete-Time Integrator1 : DiscreteIntegrator  SampleTime=0.01  ICPrevOutput=DiscIntNeverNeededParam  ICPrevScaledInput=DiscIntNeverNeededParam
  Discrete-Time Integrator2 : DiscreteIntegrator  SampleTime=0.01  ICPrevOutput=DiscIntNeverNeededParam  ICPrevScaledInput=DiscIntNeverNeededParam
  Discrete-Time Integrator3 : DiscreteIntegrator  SampleTime=0.01  LimitOutput=on  LowerSaturationLimit=0  ICPrevOutput=DiscIntNeverNeededParam  ICPrevScaledInput=DiscIntNeverNeededParam
  Divide : Product  Inputs=**
  E_brake : Saturate  UpperLimit=0  LowerLimit=-inf
  E_propel : Saturate  UpperLimit=inf  LowerLimit=0
  Force2Acceleration : Gain  Gain=1/inertialMassVeh
      settings: AttributesFormatString=%<Gain>
  GradeForce[N] : Constant  Value=massVeh*gravity
      settings: AttributesFormatString=%<Value>
  J2kWh : Gain  Gain=0.000278/1000
  Product : Product
  RollingResistance[N] : Constant  Value=massVeh*gravity*rollingResistCoeff
      settings: AttributesFormatString=%<Value>
  Sum : Sum  Inputs=+---
  Trigonometric Function : Trigonometry
  Vel^2 : Math  Operator=magnitude^2  SaturateOnIntegerOverflow=on
  mph2mph : Gain  Gain=2.23693629
  w2kw : Gain  Gain=0.001
  GliderOutput : Outport
  acc : Outport  Port=2
  wires:
  Discrete-Time Integrator3/1 -> mph2mph/1, Product/2, Discrete-Time Integrator1/1, Vel^2/1  "Velocity[mps]"
  AerodynamicDrag[N]1/1 -> Sum/2
  AerodynamicDrag[N]/1 -> AerodynamicDrag[N]1/1
  RollingResistance[N]/1 -> Sum/3
  Divide/1 -> Sum/4
  Trigonometric Function/1 -> Divide/2
  GradeForce[N]/1 -> Divide/1
  slope_angle[°]/1 -> Trigonometric Function/1
  Bus Creator/1 -> GliderOutput/1  "Glider"
  Product/1 -> w2kw/1, Discrete-Time Integrator2/1  "TractivePower[W]"
  tractiveForce[N]/1 -> Sum/1, Product/1  "TractiveForce[N]"
  Discrete-Time Integrator1/1 -> Bus Creator/7  "Position[m]"
  E_brake/1 -> Bus Creator/5  "BrakingEnergy[J]"
  Force2Acceleration/1 -> acc/1, Discrete-Time Integrator3/1  "Acceleration[mpss]"
  Discrete-Time Integrator2/1 -> E_propel/1, E_brake/1, Bus Creator/3, J2kWh/1  "TotalTractiveEnergy[J]"
  Vel^2/1 -> AerodynamicDrag[N]/1
  w2kw/1 -> Bus Creator/1  "TractivePower[kW]"
  E_propel/1 -> Bus Creator/4  "PropellingEnergy[J]"
  mph2mph/1 -> Bus Creator/6  "Velocity[mph]"
  Sum/1 -> Force2Acceleration/1  "InertialForce[N]"
  J2kWh/1 -> Bus Creator/2  "TotalTractiveEnergy[kWh]"

== system PCC_Calibration_Simu/vehicle_mode1/touque-acc convert ==
  note: 原先这里有一阶传递函数滤波，现在拿掉
  EngSpd : Inport
  Te_q : Inport  Port=2
  Te : Inport  Port=3
  Add1 : Sum
  Constant4 : Constant  Value=0
  Discrete PID Controller : simulink/Continuous/PID Controller  Controller=PID  TimeDomain=Discrete-time  SampleTime=0.01  IntegratorMethod=Forward Euler  FilterMethod=Forward Euler  Form=Parallel  UseFilter=on  ControllerParametersSource=internal  P=0.003  I=0.001  D=0  N=100  InitialConditionSource=internal  InitialConditionForIntegrator=0  InitialConditionForFilter=0  ExternalReset=none  LimitOutput=off  UpperSaturationLimit=inf  LowerSaturationLimit=-inf  LinearizeAsGain=off  AntiWindupMode=none  Kb=1  TrackingMode=off  Kt=1  PParamMin=[]  PParamMax=[]  IParamMin=[]  IParamMax=[]  DParamMin=[]  DParamMax=[]  NParamMin=[]  NParamMax=[]  KbParamMin=[]  KbParamMax=[]  KtParamMin=[]  KtParamMax=[]  POutMin=[]  POutMax=[]  IOutMin=[]  IOutMax=[]  DOutMin=[]  DOutMax=[]  NOutMin=[]  NOutMax=[]  KbOutMin=[]  KbOutMax=[]  KtOutMin=[]  KtOutMax=[]  IntegratorOutMin=[]  IntegratorOutMax=[]  FilterOutMin=[]  FilterOutMax=[]  SumOutMin=[]  SumOutMax=[]  SumI1OutMin=[]  SumI1OutMax=[]  SumI2OutMin=[]  SumI2OutMax=[]  SumI3OutMin=[]  SumI3OutMax=[]  SumDOutMin=[]  SumDOutMax=[]  SaturationOutMin=[]  SaturationOutMax=[]  IntegratorContinuousStateAttributes=''  IntegratorStateMustResolveToSignalObject=off  IntegratorRTWStateStorageClass=Auto  FilterContinuousStateAttributes=''  FilterStateMustResolveToSignalObject=off  FilterRTWStateStorageClass=Auto  DifferentiatorICPrevScaledInput=0  DifferentiatorOutMin=[]  DifferentiatorOutMax=[]
  Gain2 : Gain
  Memory : Memory  InheritSampleTime=on
  Saturation : Saturate  UpperLimit=6700  LowerLimit=700
  Saturation1 : Saturate  UpperLimit=1  LowerLimit=0
  Sum2 : Sum  Inputs=|+-
  Switch2 : Switch  Threshold=0.1
  engine inverse MAP : Lookup2D  RowIndex=speed  ColumnIndex=Te  Table=z_ACCe  InputSameDT=on
  radstorpm : Gain  Gain=9.5488095
  acc_e : Outport
  wires:
  Memory/1 -> Sum2/2
  radstorpm/1 -> Saturation/1
  EngSpd/1 -> radstorpm/1
  engine inverse MAP/1 -> Gain2/1
  Gain2/1 -> Add1/1
  Switch2/1 -> acc_e/1
  Constant4/1 -> Switch2/3
  [Te_q] -> Switch2/2
  Te_q/1 -> Sum2/1, engine inverse MAP/2, [Te_q]
  Te/1 -> Memory/1
  Saturation1/1 -> Switch2/1
  Saturation/1 -> engine inverse MAP/1
  Sum2/1 -> Discrete PID Controller/1
  Add1/1 -> Saturation1/1
  Discrete PID Controller/1 -> Add1/2

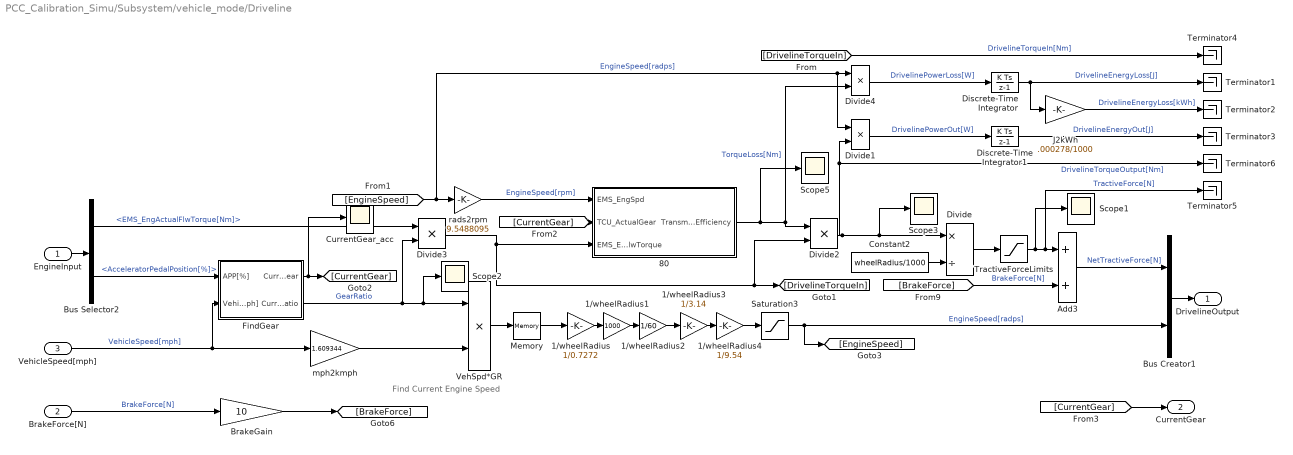
== system PCC_Calibration_Simu/Subsystem/vehicle_mode/Driveline ==
  note: Find Current Engine Speed
  EngineInput : Inport
  BrakeForce[N] : Inport  Port=2
  VehicleSpeed[mph] : Inport  Port=3
  1/wheelRadius : Gain  Gain=1/0.7272
  1/wheelRadius1 : Gain  Gain=1000
  1/wheelRadius2 : Gain  Gain=1/60
  1/wheelRadius3 : Gain  Gain=1/3.14
  1/wheelRadius4 : Gain  Gain=1/9.54
  80 : Subsystem
  Add3 : Sum
  BrakeGain : Gain  Gain=10
  Bus Creator1 : BusCreator  Inputs=2
  Bus Selector2 : BusSelector  OutputSignals=EMS_EngActualFlwTorque[Nm],AcceleratorPedalPosition[%]
  Constant2 : Constant  Value=wheelRadius/1000
  CurrentGear_acc : Scope
  Discrete-Time Integrator : DiscreteIntegrator  SampleTime=0.01  ICPrevOutput=DiscIntNeverNeededParam  ICPrevScaledInput=DiscIntNeverNeededParam
  Discrete-Time Integrator1 : DiscreteIntegrator  SampleTime=0.01  ICPrevOutput=DiscIntNeverNeededParam  ICPrevScaledInput=DiscIntNeverNeededParam
  Divide : Product  Inputs=*/
  Divide{1..4} (4 alike) : Product  Inputs=**
  FindGear : Subsystem
  J2kWh : Gain  Gain=.000278/1000
  Memory : Memory  InheritSampleTime=on
  Saturation3 : Saturate  UpperLimit=inf  LowerLimit=0.001  ZeroCross=off
  Scope{1..3,5} (4 alike) : Scope
  Terminator{1..6} (6 alike) : Terminator
  TractiveForceLimits : Saturate  UpperLimit=MDL.DrivelineModel.Ftr_max  LowerLimit=0  ZeroCross=off
  VehSpd*GR : Product  Inputs=**
  mph2kmph : Gain  Gain=1.609344
  rads2rpm : Gain  Gain=9.5488095
  DrivelineOutput : Outport
  CurrentGear : Outport  Port=2
  wires:
  Divide2/1 -> Terminator6/1, Divide1/2, Scope3/1, Divide/1  "DrivelineTorqueOutput[Nm]"
  Divide/1 -> TractiveForceLimits/1
  [BrakeForce] -> Add3/2  "BrakeForce[N]"
  TractiveForceLimits/1 -> Scope1/1, Terminator5/1, Add3/1  "TractiveForce[N]"
  EngineInput/1 -> Bus Selector2/1
  Add3/1 -> Bus Creator1/1  "NetTractiveForce[N]"
  Saturation3/1 -> [EngineSpeed], Bus Creator1/2  "EngineSpeed[radps]"
  FindGear/2(CurrentGearRatio) -> Divide3/2, Scope2/1, VehSpd*GR/1  "GearRatio"
  Constant2/1 -> Divide/2
  Bus Selector2/1 -> Divide3/1  "<EMS_EngActualFlwTorque[Nm]>"
  Divide3/1 -> 80/3(EMS_EngActualFlwTorque), Divide2/2, [DrivelineTorqueIn]
  Divide4/1 -> Discrete-Time Integrator/1  "DrivelinePowerLoss[W]"
  [EngineSpeed] -> rads2rpm/1, Divide1/1, Divide4/1  "EngineSpeed[radps]"
  Divide1/1 -> Discrete-Time Integrator1/1  "DrivelinePowerOut[W]"
  Discrete-Time Integrator1/1 -> Terminator3/1  "DrivelineEnergyOut[J]"
  J2kWh/1 -> Terminator2/1  "DrivelineEnergyLoss[kWh]"
  Discrete-Time Integrator/1 -> J2kWh/1, Terminator1/1  "DrivelineEnergyLoss[J]"
  Bus Selector2/2 -> FindGear/1(APP[%])  "<AcceleratorPedalPosition[%]>"
  80/1(TransmissionEfficiency) -> Scope5/1, Divide4/2, Divide2/1  "TorqueLoss[Nm]"
  rads2rpm/1 -> 80/1(EMS_EngSpd)  "EngineSpeed[rpm]"
  Bus Creator1/1 -> DrivelineOutput/1
  [DrivelineTorqueIn] -> Terminator4/1  "DrivelineTorqueIn[Nm]"
  BrakeForce[N]/1 -> BrakeGain/1  "BrakeForce[N]"
  VehicleSpeed[mph]/1 -> mph2kmph/1, FindGear/2(VehicleSpeed[mph])  "VehicleSpeed[mph]"
  BrakeGain/1 -> [BrakeForce]
  FindGear/1(CurrentGear) -> CurrentGear_acc/1, [CurrentGear]
  [CurrentGear] -> 80/2(TCU_ActualGear)
  1/wheelRadius/1 -> 1/wheelRadius1/1
  mph2kmph/1 -> VehSpd*GR/2
  1/wheelRadius1/1 -> 1/wheelRadius2/1
  1/wheelRadius2/1 -> 1/wheelRadius3/1
  1/wheelRadius3/1 -> 1/wheelRadius4/1
  1/wheelRadius4/1 -> Saturation3/1
  [CurrentGear] -> CurrentGear/1
  VehSpd*GR/1 -> Memory/1
  Memory/1 -> 1/wheelRadius/1

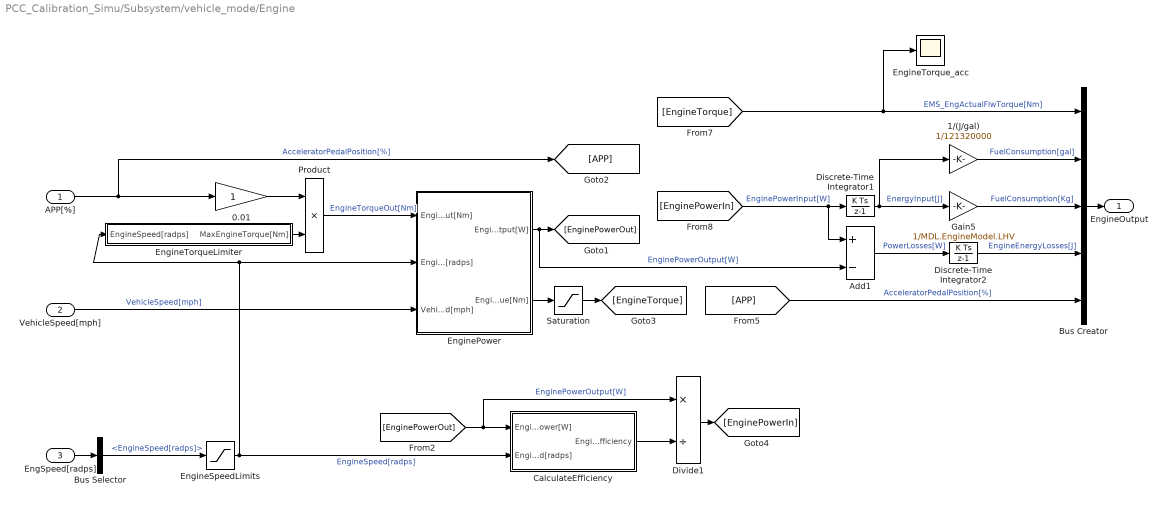
== system PCC_Calibration_Simu/Subsystem/vehicle_mode/Engine ==
  APP[%] : Inport
  VehicleSpeed[mph] : Inport  Port=2
  EngSpeed[radps] : Inport  Port=3
  0.01 : Gain
  1/(J/gal) : Gain  Gain=1/121320000
  Add1 : Sum  Inputs=+-
  Bus Creator : BusCreator  Inputs=5
  Bus Selector : BusSelector  OutputSignals=EngineSpeed[radps]
  CalculateEfficiency : Subsystem
  Discrete-Time Integrator1 : DiscreteIntegrator  SampleTime=0.01  ICPrevOutput=DiscIntNeverNeededParam  ICPrevScaledInput=DiscIntNeverNeededParam
  Discrete-Time Integrator2 : DiscreteIntegrator  SampleTime=0.01  ICPrevOutput=DiscIntNeverNeededParam  ICPrevScaledInput=DiscIntNeverNeededParam
  Divide1 : Product  Inputs=*/
  EnginePower : Subsystem
  EngineSpeedLimits : Saturate  UpperLimit=940  LowerLimit=84
  EngineTorqueLimiter : Subsystem
  EngineTorque_acc : Scope
  Gain5 : Gain  Gain=1/MDL.EngineModel.LHV
      settings: AttributesFormatString=%<Gain>
  Product : Product  RndMeth=Zero
  Saturation : Saturate  UpperLimit=120  LowerLimit=0
  EngineOutput : Outport
  wires:
  APP[%]/1 -> [APP], 0.01/1  "AcceleratorPedalPosition[%]"
  0.01/1 -> Product/1
  Discrete-Time Integrator1/1 -> Gain5/1, 1/(J/gal)/1  "EnergyInput[J]"
  Bus Creator/1 -> EngineOutput/1
  1/(J/gal)/1 -> Bus Creator/2  "FuelConsumption[gal]"
  Discrete-Time Integrator2/1 -> Bus Creator/4  "EngineEnergyLosses[J]"
  Gain5/1 -> Bus Creator/3  "FuelConsumption[Kg]"
  EngSpeed[radps]/1 -> Bus Selector/1
  CalculateEfficiency/1(EngineEfficiency) -> Divide1/2
  Add1/1 -> Discrete-Time Integrator2/1  "PowerLosses[W]"
  [APP] -> Bus Creator/5  "AcceleratorPedalPosition[%]"
  EngineTorqueLimiter/1(MaxEngineTorque[Nm]) -> Product/2
  Product/1 -> EnginePower/1(EngineTorqueOut[Nm])  "EngineTorqueOut[Nm]"
  EngineSpeedLimits/1 -> EnginePower/2(EngineSpeed[radps]), EngineTorqueLimiter/1(EngineSpeed[radps]), CalculateEfficiency/2("EngineSpeed[radps] ")  "EngineSpeed[radps]"
  VehicleSpeed[mph]/1 -> EnginePower/3(VehicleSpeed[mph])  "VehicleSpeed[mph]"
  Bus Selector/1 -> EngineSpeedLimits/1  "<EngineSpeed[radps]>"
  [EnginePowerOut] -> Divide1/1, CalculateEfficiency/1(EnginePower[W])  "EnginePowerOutput[W]"
  EnginePower/1(EnginePowerOutput[W]) -> [EnginePowerOut], Add1/2  "EnginePowerOutput[W]"
  EnginePower/2(EngineTorque[Nm]) -> Saturation/1
  [EngineTorque] -> EngineTorque_acc/1, Bus Creator/1  "EMS_EngActualFlwTorque[Nm]"
  Divide1/1 -> [EnginePowerIn]
  [EnginePowerIn] -> Discrete-Time Integrator1/1, Add1/1  "EnginePowerInput[W]"
  Saturation/1 -> [EngineTorque]
